simulink model "DC_Motor_BrakeMode"  (R2018a)
settings: Solver=VariableStepAuto  StartTime=0.0  StopTime=10.0  FixedStep=1e-5  RelTol=1e-3
PreLoadFcn:
  | modelDir = fileparts(get_param(bdroot, 'FileName'));
  | addpath(fullfile(modelDir,'Parameters'));
  | addpath(fullfile(modelDir,'subsystems'));
  | 
  | Parameters_Model
  | Parameters_Simulation
  | Parameters_Controller
InitFcn:
  | Parameters_Model
  | Parameters_Simulation
  | Parameters_Controller
undefined symbols (not defined in the file): B, dTheta0, I0, J, Ke, Kt, L, R, theta0
settings Model: Creator=Thomas  LastModifiedBy=Thomas

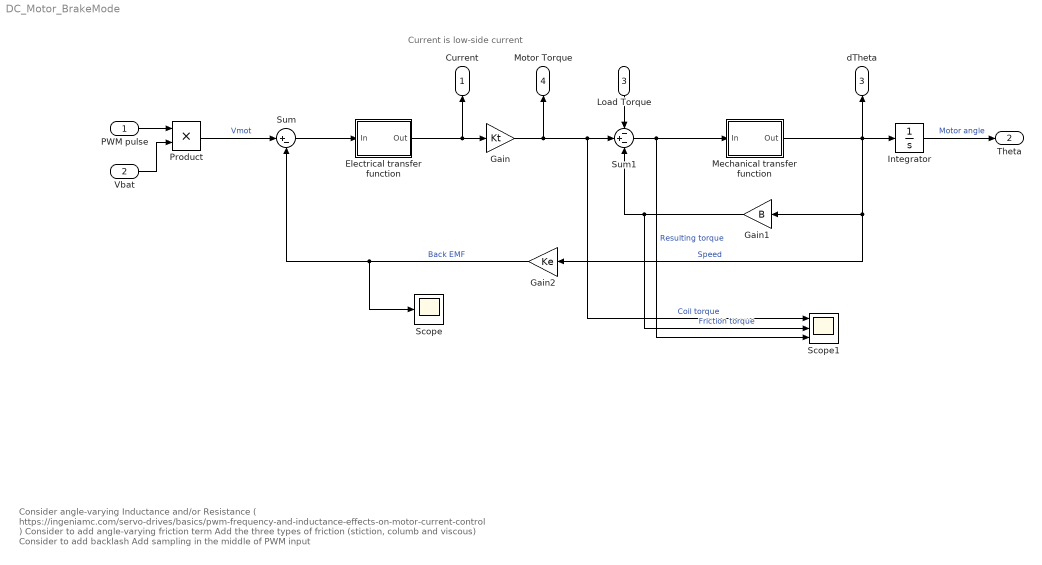
== system DC_Motor_BrakeMode ==
  note: Consider angle-varying Inductance and/or Resistance ( https://ingeniamc.com/servo-drives/basics/pwm-frequency-and-inductance-effects-on-motor-current-control )
      | Consider to add angle-varying friction term
      | Add the three types of friction (stiction, columb and viscous)
      | Consider to add backlash
      | Add sampling in the middle of PWM input
  note: Current is low-side current
  PWM pulse : Inport  OutDataTypeStr=boolean
  Vbat : Inport  Port=2  OutDataTypeStr=double
  Load Torque : Inport  Port=3  OutDataTypeStr=double
  Electrical transfer function : Subsystem
  Gain : Gain  Gain=Kt
  Gain1 : Gain  Gain=B
  Gain2 : Gain  Gain=Ke
  Integrator : Integrator  InitialCondition=theta0
  Mechanical transfer function : Subsystem
  Product : Product
  Scope : Scope
  Scope1 : Scope  NumInputPorts=3
  Sum : Sum  Inputs=|+-
  Sum1 : Sum  Inputs=-+-
  Current : Outport
  Theta : Outport  Port=2
  dTheta : Outport  Port=3
  Motor Torque : Outport  Port=4
  wires:
  Vbat/1 -> Product/2
  PWM pulse/1 -> Product/1
  Product/1 -> Sum/1  "Vmot"
  Electrical transfer function/1(Out) -> Current/1, Gain/1
  Sum/1 -> Electrical transfer function/1(In)
  Gain/1 -> Scope1/1, Sum1/2, Motor Torque/1  "Coil torque"
  Load Torque/1 -> Sum1/1
  Sum1/1 -> Mechanical transfer function/1(In), Scope1/3  "Resulting torque"
  Mechanical transfer function/1(Out) -> Gain2/1, Gain1/1, Integrator/1, dTheta/1  "Speed"
  Gain1/1 -> Scope1/2, Sum1/3  "Friction torque"
  Integrator/1 -> Theta/1  "Motor angle"
  Gain2/1 -> Scope/1, Sum/2  "Back EMF"

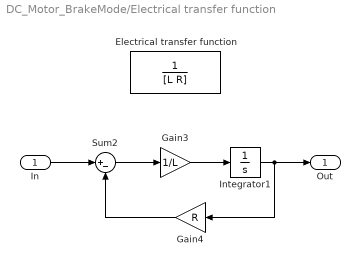
== system DC_Motor_BrakeMode/Electrical transfer function ==
  In : Inport
  Electrical transfer function : TransferFcn  Denominator=[L R]
  Gain3 : Gain  Gain=1/L
  Gain4 : Gain  Gain=R
  Integrator1 : Integrator  InitialCondition=I0
  Sum2 : Sum  Inputs=|+-
  Out : Outport
  wires:
  In/1 -> Sum2/1
  Gain3/1 -> Integrator1/1
  Gain4/1 -> Sum2/2
  Sum2/1 -> Gain3/1
  Integrator1/1 -> Out/1, Gain4/1

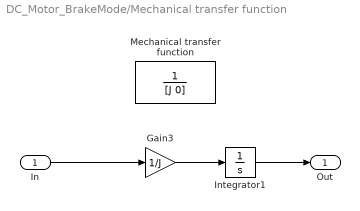
== system DC_Motor_BrakeMode/Mechanical transfer function ==
  In : Inport
  Gain3 : Gain  Gain=1/J
  Integrator1 : Integrator  InitialCondition=dTheta0
  Mechanical transfer function : TransferFcn  Denominator=[J 0]
  Out : Outport
  wires:
  Gain3/1 -> Integrator1/1
  In/1 -> Gain3/1
  Integrator1/1 -> Out/1
